simulink model "FM_Tx_Rx_Baseband_Sine"  (R2026a)
settings: Solver=VariableStepAuto  StopTime=2
model workspace (MAT data in the model file):
  FrameSize = 1000
  Fs = 100000
  Kf = 2000
libraries: commanabbnd3 x2, commchan3 x1, dspsigops x1, dspfdesign x1, dspsrcs4 x1, commrflib2 x1
settings Model: Creator=ranja  LastModifiedBy=ranja

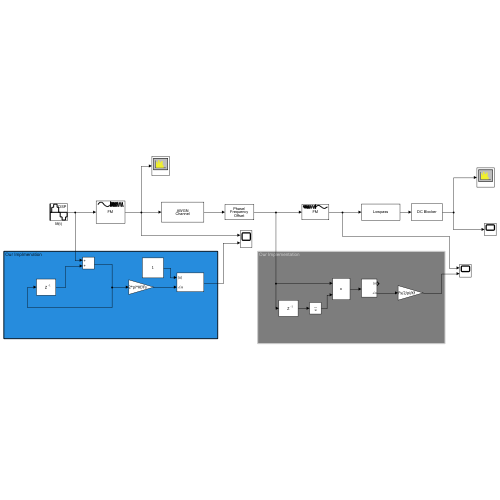
[thumbnail: Simulink's stored preview of the top-level diagram]
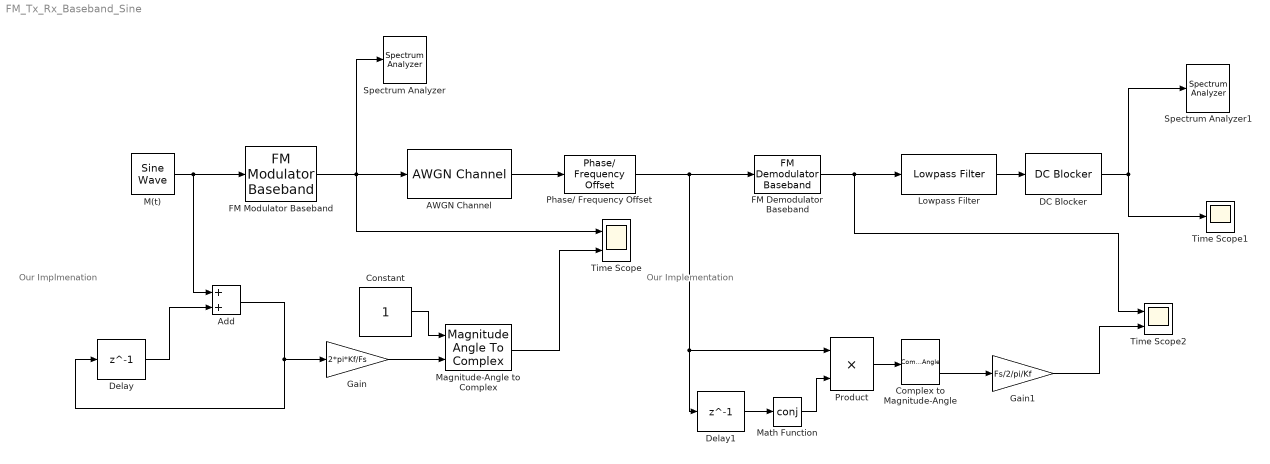
== system FM_Tx_Rx_Baseband_Sine ==
  note: Our Implementation
  note: Our Implmenation
  AWGN Channel : commchan3/AWGN Channel  LegacyMode=off  NoiseMethod="Signal to noise ratio  (SNR)"  noiseMode="Signal to noise ratio  (SNR)"  EbNo=10  EsNo=10  SNR=20  BitsPerSymbol=1  SignalPower=1  SpecifySymbolPeriod=off  SamplesPerSymbol=1  SymbolPeriod=1  VarianceSource=Parameter  Variance=1  RandomStream=Global stream  Seed=67  SimulateUsing=Code generation
  Add : Sum
  Complex to Magnitude-Angle : ComplexToMagnitudeAngle
  Constant : Constant
  DC Blocker : dspsigops/DC Blocker  Algorithm=IIR  NormalizedBandwidth=0.001  Length=8  Order=6  SimulateUsing=Code generation
      settings: LibrarySourceBlock=commhdlfilt/DC Blocker
  Delay : Delay  DelayLength=1
  Delay1 : Delay  DelayLength=1
  "FM Demodulator Baseband " : commanabbnd3/FM Demodulator Baseband   FrequencyDeviation=Kf  SimulateUsing=Code generation
  FM Modulator Baseband : commanabbnd3/FM Modulator Baseband  FrequencyDeviation=Kf  SimulateUsing=Code generation
  Gain : Gain  Gain=2*pi*Kf/Fs
  Gain1 : Gain  Gain=Fs/2/pi/Kf
  Lowpass Filter : dspfdesign/Lowpass Filter  FilterType=FIR  DesignForMinimumOrder=off  FilterOrder=50  PassbandFrequency=150  StopbandFrequency=0.5442  PassbandRipple=0.1  StopbandAttenuation=80  SampleRateMode=Specify on dialog  SampleRate=Fs  SimulateUsing=Interpreted execution  roundingMode=Floor  coeffsDataTypeStr=fixdt(1,16)
  M(t) : dspsrcs4/Sine Wave  Amplitude=1  Frequency=100  Phase=0  SampleMode=Discrete  OutComplex=Real  CompMethod=Trigonometric fcn  TableSize=Speed  SampleTime=1/Fs  SamplesPerFrame=FrameSize  ResetState=Restart at time zero  OutputFrames=off  dataType=double  wordLen=16  udDataType=sfix(16)  fracBitsMode=Best precision  numFracBits=15  OutDataTypeStr=double  LastOutDataTypeStr=double
  Magnitude-Angle to Complex : MagnitudeAngleToComplex
  Math Function : Math  Operator=conj
  Phase/ Frequency Offset : commrflib2/Phase// Frequency Offset  PhaseOffset=30  FrequencyOffsetFromPort=off  FrequencyOffset=350  SimulateUsing=Code generation
  Product : Product
  Spectrum Analyzer : SpectrumAnalyzer  WindowPosition=[1.000000,49.000000,1536.000000,793.000000,]  ScopeFrameLocation=window  WindowInvariantSamplesPerUpdate=on  Span=100000  StartFrequency=-50000  StopFrequency=50000  YLimits=[-133.5122 32.9507]
  Spectrum Analyzer1 : SpectrumAnalyzer  WindowPosition=[1.000000,49.000000,1536.000000,793.000000,]  ScopeFrameLocation=window  WindowInvariantSamplesPerUpdate=on  FrequencySpan=Span and center frequency  Span=5000  YLimits=[-46.8433 27.6752]  SelectedToolstripTab=spectrumAnalyzerToolstrip.estimationTab
  Time Scope : Scope  NumInputPorts=2
      settings: TimeUnits=Metric (based on Time Span)  ActiveDisplayYMinimum=-1.1650896571688834  ActiveDisplayYMaximum=1.1362800165577553  YLabel=Amplitude
  Time Scope1 : Scope
      settings: TimeUnits=Metric (based on Time Span)  ActiveDisplayYMinimum=-0.9979553181174925  ActiveDisplayYMaximum=1.272679151484247  YLabel=Amplitude
  Time Scope2 : Scope  NumInputPorts=2
      settings: TimeUnits=Metric (based on Time Span)  ActiveDisplayYMinimum=-1.1650896571688834  ActiveDisplayYMaximum=1.1362800165577553  YLabel=Amplitude  DataLoggingVariableName=ScopeData2
  wires:
  FM Modulator Baseband/1 -> AWGN Channel/1, Time Scope/1, Spectrum Analyzer/1
  M(t)/1 -> Add/1, FM Modulator Baseband/1
  AWGN Channel/1 -> Phase/ Frequency Offset/1
  Phase/ Frequency Offset/1 -> Delay1/1, Product/1, "FM Demodulator Baseband "/1
  "FM Demodulator Baseband "/1 -> Time Scope2/1, Lowpass Filter/1
  Lowpass Filter/1 -> DC Blocker/1
  DC Blocker/1 -> Time Scope1/1, Spectrum Analyzer1/1
  Add/1 -> Delay/1, Gain/1
  Delay/1 -> Add/2
  Gain/1 -> Magnitude-Angle to Complex/2
  Constant/1 -> Magnitude-Angle to Complex/1
  Magnitude-Angle to Complex/1 -> Time Scope/2
  Delay1/1 -> Math Function/1
  Math Function/1 -> Product/2
  Product/1 -> Complex to Magnitude-Angle/1
  Complex to Magnitude-Angle/2 -> Gain1/1
  Gain1/1 -> Time Scope2/2
